simulink library "active_model"  (R2018a)
settings: Solver=VariableStepAuto  StartTime=0.0  StopTime=10.0  RelTol=1e-3
values from neighbouring files (symbols this model uses):
  c = 1000    [parameters.m]
  k = 16812    [parameters.m]
  kt = 190000    [parameters.m]
  ms = 105    [parameters.m]
  mu = 50    [parameters.m]
libraries: simulink x5, sdolib x1
settings Model: Creator=Saurabh Suman  LastModifiedBy=Saurabh Suman

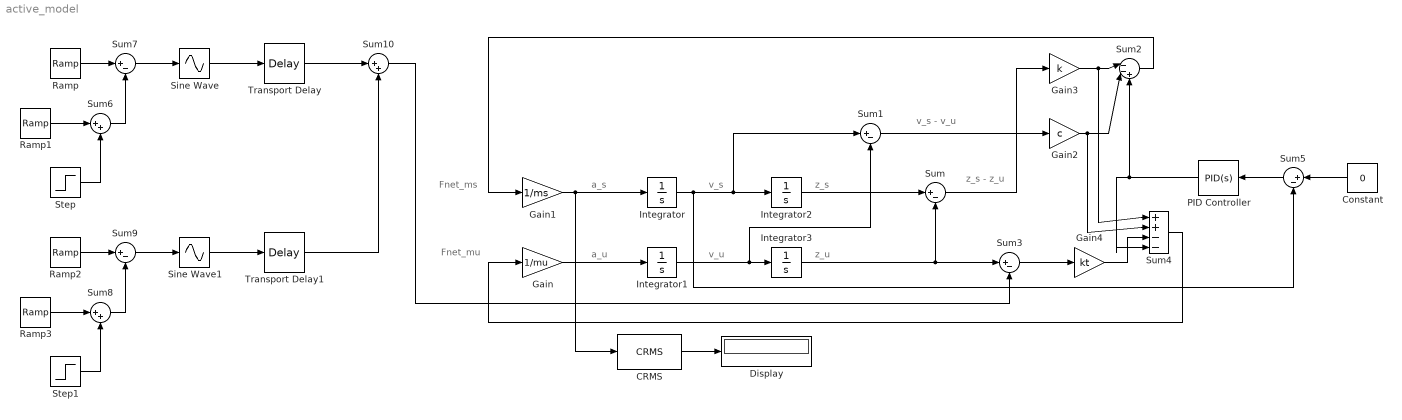
== system active_model ==
  note: z_s - z_u
  note: v_s - v_u
  note: Fnet_mu
  note: Fnet_ms
  note: a_u
  note: z_u
  note: z_s
  note: a_s
  note: v_s
  note: v_u
  CRMS : sdolib/RMS Blocks/CRMS
      settings: SourceProductName=Simulink Design Optimization  SourceProductBaseCode=SO
  Constant : Constant  Value=0
  Display : Display
  Gain : Gain  Gain=1/mu
  Gain1 : Gain  Gain=1/ms
  Gain2 : Gain  Gain=c
  Gain3 : Gain  Gain=k
  Gain4 : Gain  Gain=kt
  Integrator{,1..3} (4 alike) : Integrator
  PID Controller : simulink/Continuous/PID Controller  Controller=PID  TimeDomain=Continuous-time  SampleTime=-1  IntegratorMethod=Forward Euler  FilterMethod=Forward Euler  Form=Parallel  UseFilter=on  ControllerParametersSource=internal  P=1  I=1  D=0  N=100  InitialConditionSource=internal  InitialConditionForIntegrator=0  InitialConditionForFilter=0  ExternalReset=none  LimitOutput=off  UpperSaturationLimit=inf  LowerSaturationLimit=-inf  LinearizeAsGain=on  AntiWindupMode=none  Kb=1  TrackingMode=off  Kt=1  PParamMin=[]  PParamMax=[]  IParamMin=[]  IParamMax=[]  DParamMin=[]  DParamMax=[]  NParamMin=[]  NParamMax=[]  KbParamMin=[]  KbParamMax=[]  KtParamMin=[]  KtParamMax=[]  POutMin=[]  POutMax=[]  IOutMin=[]  IOutMax=[]  DOutMin=[]  DOutMax=[]  NOutMin=[]  NOutMax=[]  KbOutMin=[]  KbOutMax=[]  KtOutMin=[]  KtOutMax=[]  IntegratorOutMin=[]  IntegratorOutMax=[]  FilterOutMin=[]  FilterOutMax=[]  SumOutMin=[]  SumOutMax=[]  SumI1OutMin=[]  SumI1OutMax=[]  SumI2OutMin=[]  SumI2OutMax=[]  SumI3OutMin=[]  SumI3OutMax=[]  SumDOutMin=[]  SumDOutMax=[]  SaturationOutMin=[]  SaturationOutMax=[]  IntegratorContinuousStateAttributes=''  IntegratorStateMustResolveToSignalObject=off  IntegratorRTWStateStorageClass=Auto  FilterContinuousStateAttributes=''  FilterStateMustResolveToSignalObject=off  FilterRTWStateStorageClass=Auto  DifferentiatorICPrevScaledInput=0  DifferentiatorOutMin=[]  DifferentiatorOutMax=[]  FilterDiffOutCoefMin=[]  FilterDiffOutCoefMax=[]  SumDenOutMin=[]  SumDenOutMax=[]  SumNumOutMin=[]  SumNumOutMax=[]  ReciprocalOutMin=[]  ReciprocalOutMax=[]  DivideOutMin=[]  DivideOutMax=[]  TunerSelectOption=Transfer Function Based (PID Tuner App)
  Ramp : simulink/Sources/Ramp  slope=1  start=0  InitialOutput=0
  Ramp1 : simulink/Sources/Ramp  slope=1  start=1.75  InitialOutput=0
  Ramp2 : simulink/Sources/Ramp  slope=1  start=0  InitialOutput=0
  Ramp3 : simulink/Sources/Ramp  slope=1  start=1.75  InitialOutput=0
  Sine Wave : Sin  TimeSource=Use external signal  Amplitude=0.08  Frequency=1.7953  SampleTime=0
  Sine Wave1 : Sin  TimeSource=Use external signal  Amplitude=0.05  Frequency=1.7953  SampleTime=0
  Step : Step  Time=1.75  After=1.75  SampleTime=0
  Step1 : Step  Time=1.75  After=1.75  SampleTime=0
  Sum{,1,3,5,7,9} (6 alike) : Sum  Inputs=|+-
  Sum10 : Sum  Inputs=|++
  Sum2 : Sum  Inputs=|--+
  Sum4 : Sum  Inputs=|++--
  Sum6 : Sum  Inputs=|++
  Sum8 : Sum  Inputs=|++
  Transport Delay : TransportDelay  DelayTime=10
  Transport Delay1 : TransportDelay  DelayTime=30
  wires:
  Integrator/1 -> Sum5/2, Sum1/1, Integrator2/1
  Integrator1/1 -> Sum1/2, Integrator3/1
  Integrator2/1 -> Sum/1
  Gain1/1 -> CRMS/1, Integrator/1
  Gain/1 -> Integrator1/1
  Integrator3/1 -> Sum3/1, Sum/2
  Sum2/1 -> Gain1/1
  Sum4/1 -> Gain/1
  Sum1/1 -> Gain2/1
  Sum/1 -> Gain3/1
  Gain3/1 -> Sum4/1, Sum2/1
  Gain2/1 -> Sum4/2, Sum2/2
  Sum3/1 -> Gain4/1
  Gain4/1 -> Sum4/3
  PID Controller/1 -> Sum2/3, Sum4/4
  Sum5/1 -> PID Controller/1
  Constant/1 -> Sum5/1
  Ramp3/1 -> Sum8/1
  Sine Wave1/1 -> Transport Delay1/1
  Ramp2/1 -> Sum9/1
  Step1/1 -> Sum8/2
  Sum9/1 -> Sine Wave1/1
  Sum7/1 -> Sine Wave/1
  Step/1 -> Sum6/2
  Sum10/1 -> Sum3/2
  Sine Wave/1 -> Transport Delay/1
  Transport Delay1/1 -> Sum10/2
  Sum8/1 -> Sum9/2
  Ramp/1 -> Sum7/1
  Transport Delay/1 -> Sum10/1
  Sum6/1 -> Sum7/2
  Ramp1/1 -> Sum6/1
  CRMS/1 -> Display/1
